simulink model "baseline_ale"  (R2021a)
settings: Solver=FixedStepAuto  StartTime=0.0  StopTime=10.0  FixedStep=framePeriod_s  RelTol=1e-3
undefined symbols (not defined in the file or in its folder): Aircraft, analog, aux, framePeriod_s, mode, motors_enabled, pwm, sbus, throttle_cmd_prcnt, waypoint_reached
libraries: simulink x5
settings Model: Creator=brian  LastModifiedBy=remoteuser
settings SolverCC: AlgebraicLoopSolver=TrustRegion
settings OptimizationCC: DefaultParameterBehavior=Inlined  GainParamInheritBuiltInType=on  UseFloatMulNetSlope=on  DefaultUnderspecifiedDataType=single  InlineInvariantSignals=on  PassReuseOutputArgsAs=Individual arguments  ZeroExternalMemoryAtStartup=off  ZeroInternalMemoryAtStartup=off  NoFixptDivByZeroProtection=on  EfficientFloat2IntCast=on  LifeSpan=1  OptimizeBlockOrder=speed  DifferentSizesBufferReuse=on  EfficientTunableParamExpr=on
settings DebuggingCC: ParameterTunabilityLossMsg=error  SFMachineParentedDataDiag=warning
settings HardwareCC: ProdBitPerPointer=32  ProdBitPerSizeT=32  ProdBitPerPtrDiffT=32  ProdLargestAtomicInteger=Long  ProdLargestAtomicFloat=Double  ProdWordSize=32  ProdLongLongMode=on  ProdHWDeviceType=NXP->Cortex-M4
settings ModelReferenceCC: ModelReferenceNumInstancesAllowed=Single
settings SFSimCC: SimParseCustomCode=off  MATLABDynamicMemAlloc=off
settings RTWCC: SystemTargetFile=ert.tlc  GenCodeOnly=on  TemplateMakefile=ert_default_tmf  RTWVerbose=off  BuildConfiguration=Faster Runs  TargetLang=C++
settings CodeAppCC: ForceParamTrailComments=on  IgnoreCustomStorageClasses=off  OperatorAnnotations=on  SimulinkDataObjDesc=on  SFDataObjDesc=on  CustomSymbolStrGlobalVar=rt$N$M  CustomSymbolStrType=$N$M  CustomSymbolStrFcn=$N$M$F  CustomSymbolStrMacro=$N$M  InsertBlockDesc=on
settings ERTTargetCC: TargetLangStandard=C++03 (ISO)  IncludeMdlTerminateFcn=off  CombineSignalStateStructs=on  SuppressErrorStatus=on  SupportAbsoluteTime=off  CodeInterfacePackaging=C++ class  SupportNonFinite=off  SupportComplex=off  ERTHeaderFileRootName=autocode$E  ERTSourceFileRootName=autocode$E  InlinedParameterPlacement=NonHierarchical  RootIOFormat=Structure reference  ERTCustomFileTemplate=example_file_process.tlc  ERTFilePackagingFormat=Compact  ArrayContainerType=std::array

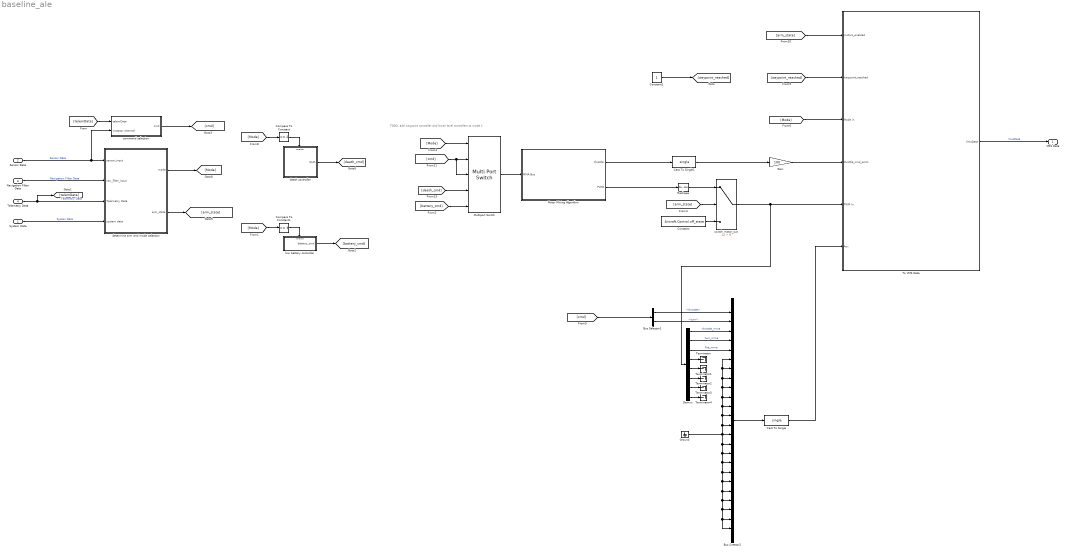
== system baseline_ale ==
  note: TODO: add waypoint controller and lower level controllers to mode 1
  System Data : Inport  OutDataTypeStr=Bus: SysData  SampleTime=framePeriod_s  BusOutputAsStruct=on
  Sensor Data : Inport  Port=2  OutDataTypeStr=Bus: SensorData  SampleTime=framePeriod_s  BusOutputAsStruct=on
  Navigation Filter Data : Inport  Port=3  OutDataTypeStr=Bus: NavData  SampleTime=framePeriod_s  BusOutputAsStruct=on
  Telemetry Data : Inport  Port=4  OutDataTypeStr=Bus: TelemData  SampleTime=framePeriod_s  BusOutputAsStruct=on
  Bus Creator2 : BusCreator  Inputs=24
  Bus Selector1 : BusSelector  OutputSignals=throttle,turn
  Cast To Single : DataTypeConversion  OutDataTypeStr=single
  Cast To Single1 : DataTypeConversion  OutDataTypeStr=single
  Compare To Constant : simulink/Logic and Bit Operations/Compare To Constant  relop===  const=2  OutDataTypeStr=boolean
  Compare To Constant1 : simulink/Logic and Bit Operations/Compare To Constant  relop===  const=3  OutDataTypeStr=boolean
  Constant : Constant  Value=Aircraft.Control.off_state  OutDataTypeStr=single  SampleTime=framePeriod_s
  Constant1 : Constant  OutDataTypeStr=boolean  SampleTime=framePeriod_s
  Demux : Demux  Outputs=8
  Gain : Gain  Gain=100
  Ground : Ground
  Motor Mixing Algorithm : Subsystem
  Multiport Switch : MultiPortSwitch  DataPortOrder=Specify indices  DataPortIndices={0, 1, 2, 3}
  Reshape : Reshape
  Terminator{,1..4} (5 alike) : Terminator
  To VMS Data : Subsystem
  command selection : Subsystem
  death controller : Subsystem
  determine arm and mode selection : Subsystem
  low battery controller : Subsystem  TreatAsAtomicUnit=on
  switch_motor_out : Switch  Criteria=u2 > Threshold
  VMS Data : Outport  OutDataTypeStr=Bus: VmsData  SampleTime=framePeriod_s  BusOutputAsStruct=on
  wires:
  [Mode] -> To VMS Data/3(Mode in)
  Gain/1 -> To VMS Data/4(throttle_cmd_prcnt)
  Reshape/1 -> switch_motor_out/1
  Bus Selector1/1 -> Bus Creator2/1  "<throttle>"
  [arm_state] -> To VMS Data/1(motors_enabled)
  Ground/1 -> Bus Creator2/20, Bus Creator2/21, Bus Creator2/24, Bus Creator2/23, Bus Creator2/22, Bus Creator2/19, Bus Creator2/18, Bus Creator2/17, Bus Creator2/16, Bus Creator2/15, Bus Creator2/6, Bus Creator2/7, Bus Creator2/8, Bus Creator2/9, Bus Creator2/10, Bus Creator2/11, Bus Creator2/12, Bus Creator2/13, Bus Creator2/14
  [waypoint_reached] -> To VMS Data/2(waypoint_reached)
  [arm_state] -> switch_motor_out/2
  switch_motor_out/1 -> Demux/1, To VMS Data/5(PWM In)
  Constant/1 -> switch_motor_out/3
  Cast To Single/1 -> To VMS Data/6(Aux)
  Bus Creator2/1 -> Cast To Single/1
  Motor Mixing Algorithm/1(throttle) -> Cast To Single1/1
  Motor Mixing Algorithm/2(PWM) -> Reshape/1
  Cast To Single1/1 -> Gain/1
  To VMS Data/1(VmsData) -> VMS Data/1  "VmsData"
  Sensor Data/1 -> command selection/2(inceptor channel), determine arm and mode selection/1(sensor_input)  "Sensor Data"
  Telemetry Data/1 -> [telemData], determine arm and mode selection/3(Telemetry Data)  "Telemetry Data"
  command selection/1(cmd) -> [cmd]
  determine arm and mode selection/1(mode) -> [Mode]
  System Data/1 -> determine arm and mode selection/4(system data)  "Systen Data"
  determine arm and mode selection/2(arm_state) -> [arm_state]
  Navigation Filter Data/1 -> determine arm and mode selection/2(nav_filter_input)  "Navigation Filter Data"
  Constant1/1 -> [waypoint_reached]
  [cmd] -> Bus Selector1/1
  Bus Selector1/2 -> Bus Creator2/2  "<turn>"
  Demux/1 -> Bus Creator2/3  "throttle_mma"
  Demux/2 -> Bus Creator2/4  "turn_mma"
  Demux/3 -> Bus Creator2/5  "fire_mma"
  Demux/4 -> Terminator/1
  Demux/5 -> Terminator1/1
  Demux/6 -> Terminator2/1
  Demux/7 -> Terminator3/1
  Demux/8 -> Terminator4/1
  [Mode] -> Multiport Switch/1
  Multiport Switch/1 -> Motor Mixing Algorithm/1(MMA Bus)
  death controller/1(Out1) -> [death_cmd]
  [Mode] -> Compare To Constant/1
  Compare To Constant/1 -> death controller/Enable
  [cmd] -> Multiport Switch/3, Multiport Switch/2
  [death_cmd] -> Multiport Switch/4
  [telemData] -> command selection/1(telemData)
  [Mode] -> Compare To Constant1/1
  Compare To Constant1/1 -> low battery controller/Enable
  low battery controller/1(battery_cmd) -> [battery_cmd]
  [battery_cmd] -> Multiport Switch/5

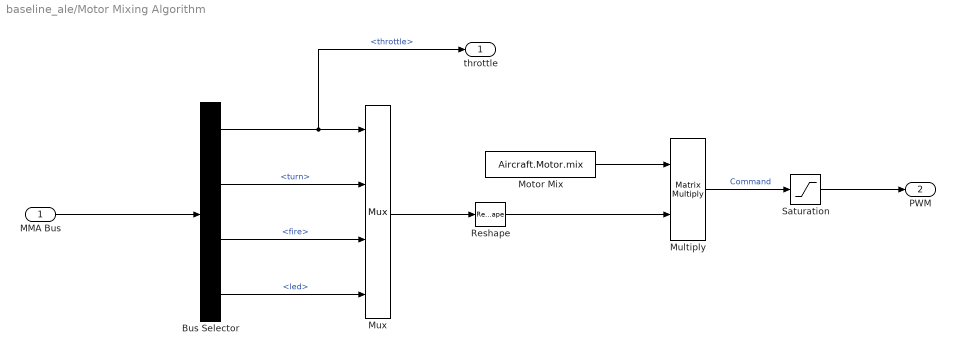
== system baseline_ale/Motor Mixing Algorithm ==
  MMA Bus : Inport
  Bus Selector : BusSelector  OutputSignals=throttle,turn,fire,led
  Motor Mix : Constant  Value=Aircraft.Motor.mix  OutDataTypeStr=single  SampleTime=framePeriod_s
  Multiply : Product  Inputs=**  Multiplication=Matrix(*)  OutDataTypeStr=single
  Mux : Mux
  Reshape : Reshape  OutputDimensionality=Column vector (2-D)
  Saturation : Saturate  UpperLimit=1  LowerLimit=-1
  throttle : Outport
  PWM : Outport  Port=2
  wires:
  Mux/1 -> Reshape/1
  MMA Bus/1 -> Bus Selector/1
  Bus Selector/1 -> Mux/1, throttle/1  "<throttle>"
  Bus Selector/2 -> Mux/2  "<turn>"
  Multiply/1 -> Saturation/1  "Command"
  Reshape/1 -> Multiply/2
  Motor Mix/1 -> Multiply/1
  Bus Selector/3 -> Mux/3  "<fire>"
  Bus Selector/4 -> Mux/4  "<led>"
  Saturation/1 -> PWM/1

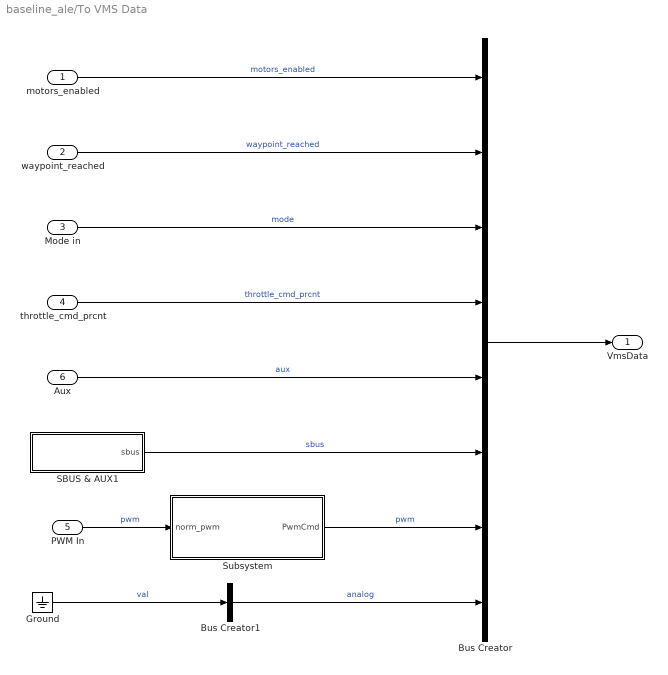
== system baseline_ale/To VMS Data ==
  motors_enabled : Inport
  waypoint_reached : Inport  Port=2
  Mode in : Inport  Port=3
  throttle_cmd_prcnt : Inport  Port=4
  PWM In : Inport  Port=5
  Aux : Inport  Port=6
  Bus Creator : BusCreator  Inputs=motors_enabled,waypoint_reached,mode,throttle_cmd_prcnt,aux,sbus,pwm,analog  OutDataTypeStr=Bus: VmsData  NonVirtualBus=on
  Bus Creator1 : BusCreator  Inputs=1  OutDataTypeStr=Bus: AnalogData
  Ground : Ground
  SBUS & AUX1 : Subsystem
  Subsystem : Subsystem
  VmsData : Outport
  wires:
  waypoint_reached/1 -> Bus Creator/2  "waypoint_reached"
  Mode in/1 -> Bus Creator/3  "mode"
  motors_enabled/1 -> Bus Creator/1  "motors_enabled"
  Bus Creator/1 -> VmsData/1
  throttle_cmd_prcnt/1 -> Bus Creator/4  "throttle_cmd_prcnt"
  PWM In/1 -> Subsystem/1(norm_pwm)  "pwm"
  Subsystem/1(PwmCmd) -> Bus Creator/7  "pwm"
  Bus Creator1/1 -> Bus Creator/8  "analog"
  Ground/1 -> Bus Creator1/1  "val"
  Aux/1 -> Bus Creator/5  "aux"
  SBUS & AUX1/1(sbus) -> Bus Creator/6  "sbus"

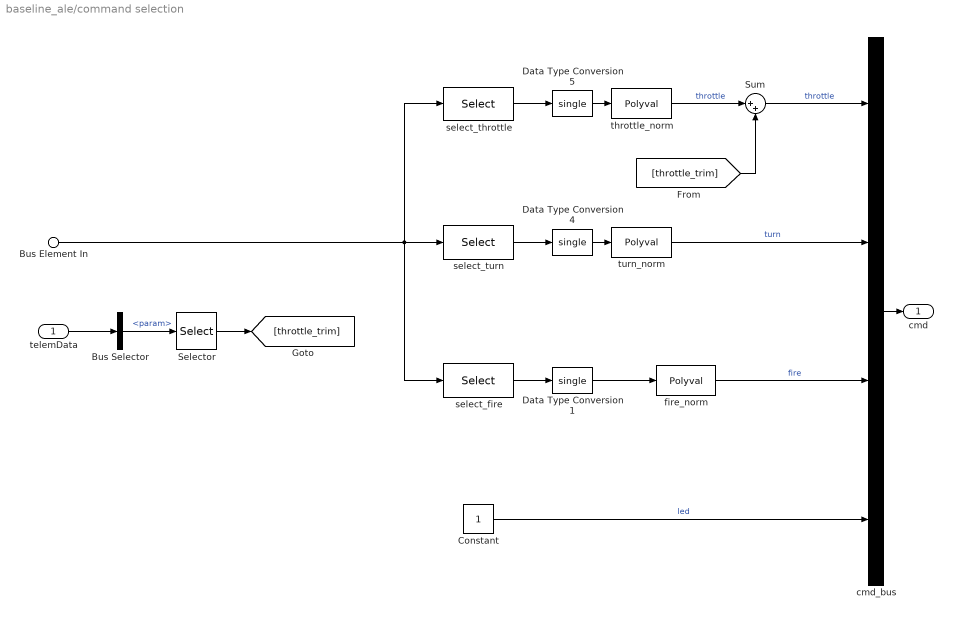
== system baseline_ale/command selection ==
  telemData : Inport
  Bus Element In : Inport  Port=2  PortName=inceptor channel  Element=inceptor.ch
  Bus Selector : BusSelector  OutputSignals=param
  Constant : Constant  OutDataTypeStr=single  SampleTime=framePeriod_s
  Data Type Conversion1 : DataTypeConversion  OutDataTypeStr=single
  Data Type Conversion4 : DataTypeConversion  OutDataTypeStr=single
  Data Type Conversion5 : DataTypeConversion  OutDataTypeStr=single
  Selector : Selector  IndexMode=Zero-based  IndexOptions=Index vector (dialog)  Indices=0  OutputSizes=1
  Sum : Sum  Inputs=|++
  cmd_bus : BusCreator  Inputs=4
  fire_norm : Polyval  Coefs=Aircraft.Inceptor.coef_2
  select_fire : Selector  IndexOptions=Index vector (dialog)  Indices=Aircraft.Inceptor.fire  OutputSizes=1
  select_throttle : Selector  IndexOptions=Index vector (dialog)  Indices=Aircraft.Inceptor.throttle  OutputSizes=1
  select_turn : Selector  IndexOptions=Index vector (dialog)  Indices=Aircraft.Inceptor.turn  OutputSizes=1
  throttle_norm : Polyval  Coefs=Aircraft.Inceptor.coef_2
  turn_norm : Polyval  Coefs=Aircraft.Inceptor.coef_2
  cmd : Outport
  wires:
  select_turn/1 -> Data Type Conversion4/1
  select_throttle/1 -> Data Type Conversion5/1
  Data Type Conversion4/1 -> turn_norm/1
  Sum/1 -> cmd_bus/1  "throttle"
  turn_norm/1 -> cmd_bus/2  "turn"
  cmd_bus/1 -> cmd/1
  Data Type Conversion5/1 -> throttle_norm/1
  Bus Element In/1 -> select_throttle/1, select_fire/1, select_turn/1
  Data Type Conversion1/1 -> fire_norm/1
  select_fire/1 -> Data Type Conversion1/1
  fire_norm/1 -> cmd_bus/3  "fire"
  Constant/1 -> cmd_bus/4  "led"
  throttle_norm/1 -> Sum/1  "throttle"
  telemData/1 -> Bus Selector/1
  Bus Selector/1 -> Selector/1  "<param>"
  Selector/1 -> [throttle_trim]
  [throttle_trim] -> Sum/2

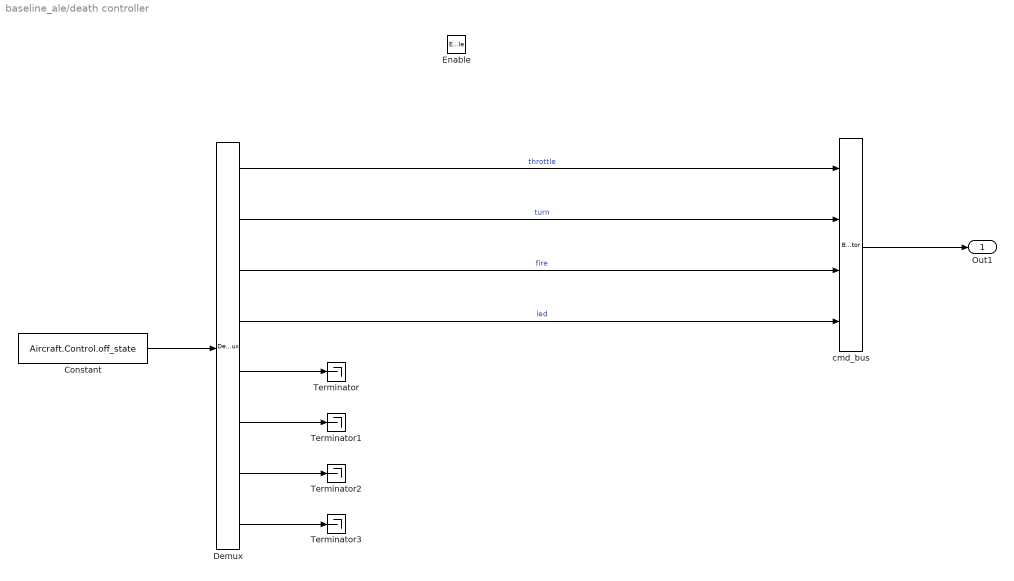
== system baseline_ale/death controller ==
  Enable : EnablePort
  Constant : Constant  Value=Aircraft.Control.off_state  OutDataTypeStr=single  SampleTime=framePeriod_s
  Demux : Demux  Outputs=8
  Terminator{,1..3} (4 alike) : Terminator
  cmd_bus : BusCreator  Inputs=4
  Out1 : Outport
  wires:
  Constant/1 -> Demux/1
  Demux/2 -> cmd_bus/2  "turn"
  Demux/3 -> cmd_bus/3  "fire"
  Demux/1 -> cmd_bus/1  "throttle"
  Demux/4 -> cmd_bus/4  "led"
  cmd_bus/1 -> Out1/1
  Demux/7 -> Terminator2/1
  Demux/8 -> Terminator3/1
  Demux/5 -> Terminator/1
  Demux/6 -> Terminator1/1

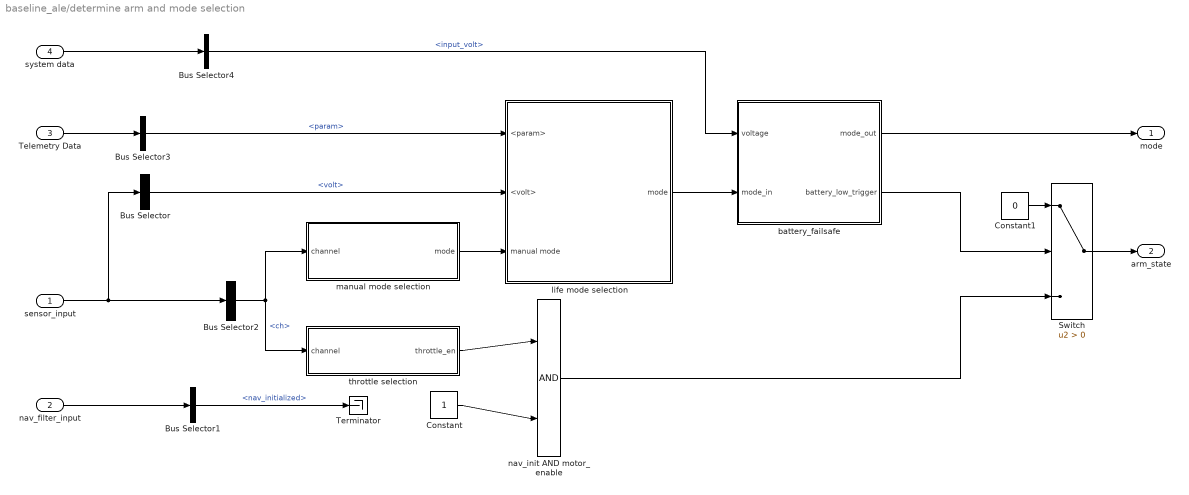
== system baseline_ale/determine arm and mode selection ==
  sensor_input : Inport
  nav_filter_input : Inport  Port=2
  Telemetry Data : Inport  Port=3
  system data : Inport  Port=4
  Bus Selector : BusSelector  OutputSignals=adc.volt
  Bus Selector1 : BusSelector  OutputSignals=nav_initialized
  Bus Selector2 : BusSelector  OutputSignals=inceptor.ch
  Bus Selector3 : BusSelector  OutputSignals=param
  Bus Selector4 : BusSelector  OutputSignals=input_volt
  Constant : Constant  OutDataTypeStr=boolean  SampleTime=framePeriod_s
  Constant1 : Constant  Value=0  OutDataTypeStr=boolean  SampleTime=framePeriod_s
  Switch : Switch  Criteria=u2 > Threshold
  Terminator : Terminator
  battery_failsafe : Subsystem
  life mode selection : Subsystem
  manual mode selection : Subsystem
  nav_init AND motor_enable : Logic  IconShape=distinctive  AllPortsSameDT=off  OutDataTypeStr=boolean
  throttle selection : Subsystem
  mode : Outport
  arm_state : Outport  Port=2
  wires:
  throttle selection/1(throttle_en) -> nav_init AND motor_enable/1
  nav_init AND motor_enable/1 -> Switch/3
  Bus Selector2/1 -> manual mode selection/1(channel), throttle selection/1(channel)  "<ch>"
  sensor_input/1 -> Bus Selector2/1, Bus Selector/1
  nav_filter_input/1 -> Bus Selector1/1
  Bus Selector1/1 -> Terminator/1  "<nav_initialized>"
  Constant/1 -> nav_init AND motor_enable/2
  Telemetry Data/1 -> Bus Selector3/1
  Bus Selector3/1 -> life mode selection/1(<param>)  "<param>"
  Bus Selector/1 -> life mode selection/2(<volt>)  "<volt>"
  manual mode selection/1(mode) -> life mode selection/3(manual mode)
  life mode selection/1(mode) -> battery_failsafe/2(mode_in)
  battery_failsafe/1(mode_out) -> mode/1
  system data/1 -> Bus Selector4/1
  Bus Selector4/1 -> battery_failsafe/1(voltage)  "<input_volt>"
  Switch/1 -> arm_state/1
  battery_failsafe/2(battery_low_trigger) -> Switch/2
  Constant1/1 -> Switch/1

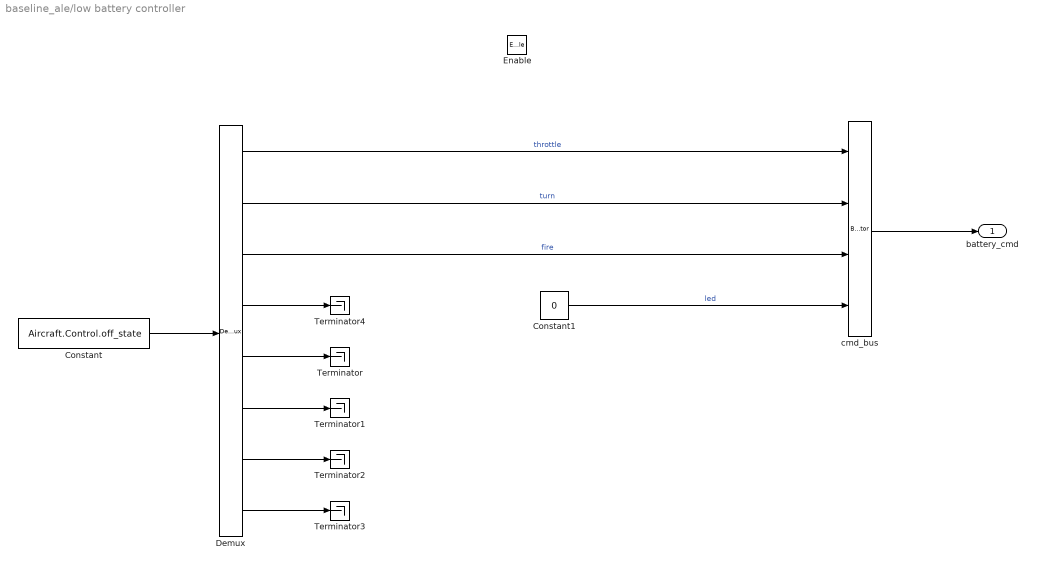
== system baseline_ale/low battery controller ==
  Enable : EnablePort
  Constant : Constant  Value=Aircraft.Control.off_state  OutDataTypeStr=single  SampleTime=framePeriod_s
  Constant1 : Constant  Value=0  OutDataTypeStr=single  SampleTime=framePeriod_s
  Demux : Demux  Outputs=8
  Terminator{,1..4} (5 alike) : Terminator
  cmd_bus : BusCreator  Inputs=4
  battery_cmd : Outport
  wires:
  Demux/5 -> Terminator/1
  Demux/7 -> Terminator2/1
  Demux/1 -> cmd_bus/1  "throttle"
  Demux/6 -> Terminator1/1
  Constant/1 -> Demux/1
  Demux/2 -> cmd_bus/2  "turn"
  Demux/8 -> Terminator3/1
  Demux/3 -> cmd_bus/3  "fire"
  cmd_bus/1 -> battery_cmd/1
  Constant1/1 -> cmd_bus/4  "led"
  Demux/4 -> Terminator4/1

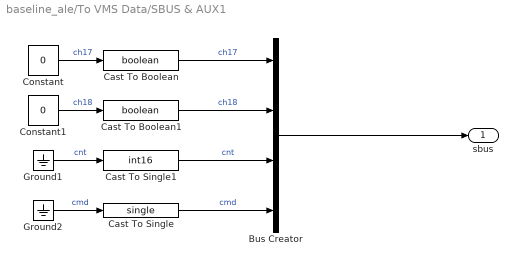
== system baseline_ale/To VMS Data/SBUS & AUX1 ==
  Bus Creator : BusCreator  Inputs=4  OutDataTypeStr=Bus: SbusCmd  NonVirtualBus=on
  Cast To Boolean : DataTypeConversion  OutDataTypeStr=boolean
  Cast To Boolean1 : DataTypeConversion  OutDataTypeStr=boolean
  Cast To Single : DataTypeConversion  OutDataTypeStr=single
  Cast To Single1 : DataTypeConversion  OutDataTypeStr=int16
  Constant : Constant  Value=0  OutDataTypeStr=boolean  SampleTime=framePeriod_s
  Constant1 : Constant  Value=0  OutDataTypeStr=boolean  SampleTime=framePeriod_s
  Ground1 : Ground
  Ground2 : Ground
  sbus : Outport  SampleTime=framePeriod_s
  wires:
  Bus Creator/1 -> sbus/1
  Constant/1 -> Cast To Boolean/1  "ch17"
  Constant1/1 -> Cast To Boolean1/1  "ch18"
  Ground2/1 -> Cast To Single/1  "cmd"
  Cast To Boolean/1 -> Bus Creator/1  "ch17"
  Cast To Boolean1/1 -> Bus Creator/2  "ch18"
  Cast To Single/1 -> Bus Creator/4  "cmd"
  Cast To Single1/1 -> Bus Creator/3  "cnt"
  Ground1/1 -> Cast To Single1/1  "cnt"

== system baseline_ale/To VMS Data/Subsystem ==
  note: cmd - output to feed to the simulator
  note: cnt - pwm output to actual hardware
  norm_pwm : Inport
  Bus Creator : BusCreator  Inputs=2  OutDataTypeStr=Bus: PwmCmd  NonVirtualBus=on
      settings: InheritFromInputs=off
  MATLAB Function : MATLAB Function  TreatAsAtomicUnit=on
  PwmCmd : Outport
  wires:
  Bus Creator/1 -> PwmCmd/1
  norm_pwm/1 -> Bus Creator/2, MATLAB Function/1(x)  "cmd"
  MATLAB Function/1(y_cnt) -> Bus Creator/1  "cnt"

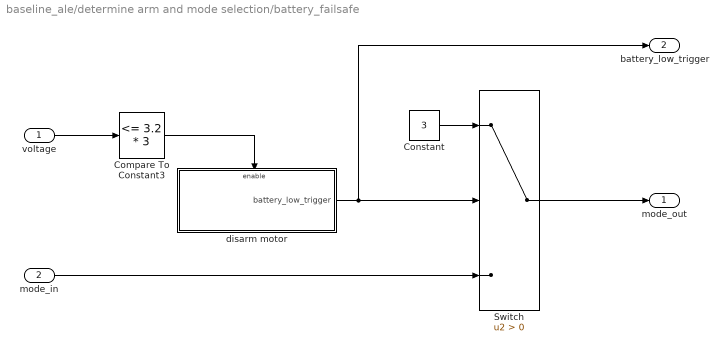
== system baseline_ale/determine arm and mode selection/battery_failsafe ==
  voltage : Inport
  mode_in : Inport  Port=2
  Compare To Constant3 : simulink/Logic and Bit Operations/Compare To Constant  relop=<=  const=3.2 * 3  OutDataTypeStr=boolean
  Constant : Constant  Value=3  OutDataTypeStr=int8  SampleTime=framePeriod_s
  Switch : Switch  Criteria=u2 > Threshold
  disarm motor : Subsystem
  mode_out : Outport
  battery_low_trigger : Outport  Port=2
  wires:
  mode_in/1 -> Switch/3
  Compare To Constant3/1 -> disarm motor/Enable
  voltage/1 -> Compare To Constant3/1
  disarm motor/1(battery_low_trigger) -> battery_low_trigger/1, Switch/2
  Switch/1 -> mode_out/1
  Constant/1 -> Switch/1

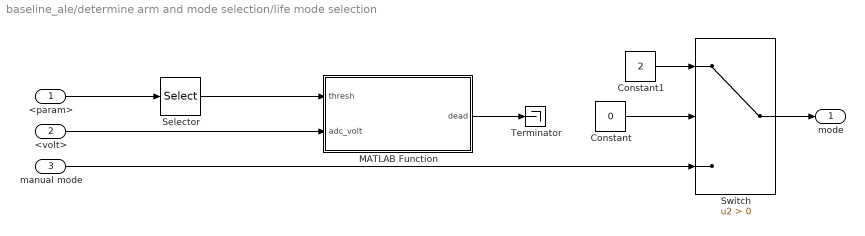
== system baseline_ale/determine arm and mode selection/life mode selection ==
  <param> : Inport
  <volt> : Inport  Port=2
  manual mode : Inport  Port=3
  Constant : Constant  Value=0  OutDataTypeStr=boolean  SampleTime=framePeriod_s
  Constant1 : Constant  Value=2  OutDataTypeStr=int8  SampleTime=framePeriod_s
  MATLAB Function : MATLAB Function  TreatAsAtomicUnit=on
  Selector : Selector  IndexMode=Zero-based  IndexOptions=Index vector (dialog)  Indices=1  OutputSizes=1
  Switch : Switch  Criteria=u2 > Threshold
  Terminator : Terminator
  mode : Outport
  wires:
  Constant1/1 -> Switch/1
  Selector/1 -> MATLAB Function/1(thresh)
  Switch/1 -> mode/1
  <param>/1 -> Selector/1
  Constant/1 -> Switch/2
  manual mode/1 -> Switch/3
  <volt>/1 -> MATLAB Function/2(adc_volt)
  MATLAB Function/1(dead) -> Terminator/1

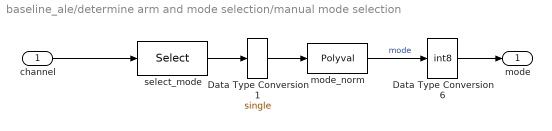
== system baseline_ale/determine arm and mode selection/manual mode selection ==
  channel : Inport
  Data Type Conversion1 : DataTypeConversion  OutDataTypeStr=single
  Data Type Conversion6 : DataTypeConversion  OutDataTypeStr=int8  RndMeth=Nearest
  mode_norm : Polyval  Coefs=Aircraft.Inceptor.coef_3
  select_mode : Selector  IndexOptions=Index vector (dialog)  Indices=Aircraft.Inceptor.mode0  OutputSizes=1
  mode : Outport
  wires:
  Data Type Conversion1/1 -> mode_norm/1
  select_mode/1 -> Data Type Conversion1/1
  mode_norm/1 -> Data Type Conversion6/1  "mode"
  Data Type Conversion6/1 -> mode/1
  channel/1 -> select_mode/1

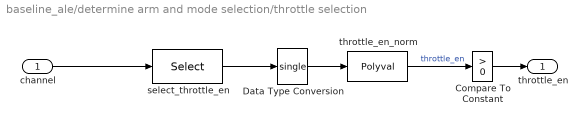
== system baseline_ale/determine arm and mode selection/throttle selection ==
  channel : Inport
  Compare To Constant : simulink/Logic and Bit Operations/Compare To Constant  relop=>  const=0  OutDataTypeStr=boolean
  Data Type Conversion : DataTypeConversion  OutDataTypeStr=single
  select_throttle_en : Selector  IndexOptions=Index vector (dialog)  Indices=Aircraft.Inceptor.throttle_en  OutputSizes=1
  throttle_en_norm : Polyval  Coefs=Aircraft.Inceptor.coef_2
  throttle_en : Outport
  wires:
  Data Type Conversion/1 -> throttle_en_norm/1
  throttle_en_norm/1 -> Compare To Constant/1  "throttle_en"
  select_throttle_en/1 -> Data Type Conversion/1
  Compare To Constant/1 -> throttle_en/1
  channel/1 -> select_throttle_en/1

== system baseline_ale/determine arm and mode selection/battery_failsafe/disarm motor ==
  Enable : EnablePort  StatesWhenEnabling=reset
  Compare To Constant2 : simulink/Logic and Bit Operations/Compare To Constant  relop=>  const=15  OutDataTypeStr=boolean
  Constant : Constant  Value=framePeriod_s
  Sum : Sum  Inputs=|++
  Unit Delay : UnitDelay  SampleTime=-1  HasFrameUpgradeWarning=on
  battery_low_trigger : Outport
  wires:
  Compare To Constant2/1 -> battery_low_trigger/1
  Sum/1 -> Compare To Constant2/1, Unit Delay/1
  Unit Delay/1 -> Sum/2
  Constant/1 -> Sum/1

== matlab function baseline_ale/To VMS Data/Subsystem/MATLAB Function ==
  data: x input; y_cnt output
function y_cnt = map_to_range(x)

y_cnt = int16((x - -1) ./ (1 - -1) .* (2000 - 1000) + 1000);

== matlab function baseline_ale/determine arm and mode selection/life mode selection/MATLAB Function ==
  data: thresh input; adc_volt input; dead output
function dead = check_alive(thresh, adc_volt)

dead = adc_volt(1) >= thresh;
